simulink model "Timers"  (R2025a)
settings: Solver=FixedStepDiscrete  StartTime=0  StopTime=1  FixedStep=1e-7  RelTol=1e-3
libraries: simulink_extras x216, simulink x13
(part 7 of 7)

== system Timers/Eg: PWM Driver+  Prescalar/Tcon/Subsystem5 ==
  Data : Inport
  Store : Inport  Port=2
  Clock : Inport  Port=3
  Clear : Inport  Port=4
  AND : Logic  IconShape=distinctive  AllPortsSameDT=off  OutDataTypeStr=boolean
  AND1 : Logic  IconShape=distinctive  AllPortsSameDT=off  OutDataTypeStr=boolean
  D Flip-Flop : simulink_extras/Flip Flops/D Flip-Flop
  NOT : Logic  Operator=NOT  IconShape=distinctive  AllPortsSameDT=off  OutDataTypeStr=boolean
  NOT1 : Logic  Operator=NOT  IconShape=distinctive  AllPortsSameDT=off  OutDataTypeStr=boolean
  OR : Logic  Operator=OR  IconShape=distinctive  AllPortsSameDT=off  OutDataTypeStr=boolean
  Q : Outport
  !Q : Outport  Port=2
  wires:
  AND1/1 -> OR/2
  AND/1 -> OR/1
  D Flip-Flop/1 -> Q/1, AND1/2
  NOT/1 -> AND1/1
  Store/1 -> AND/2, NOT/1
  Clock/1 -> D Flip-Flop/2
  Data/1 -> AND/1
  OR/1 -> D Flip-Flop/1
  D Flip-Flop/2 -> !Q/1
  Clear/1 -> NOT1/1
  NOT1/1 -> D Flip-Flop/3

== system Timers/Eg: PWM Driver+  Prescalar/Tcon/Subsystem6 ==
  Data : Inport
  Store : Inport  Port=2
  Clock : Inport  Port=3
  Clear : Inport  Port=4
  AND : Logic  IconShape=distinctive  AllPortsSameDT=off  OutDataTypeStr=boolean
  AND1 : Logic  IconShape=distinctive  AllPortsSameDT=off  OutDataTypeStr=boolean
  D Flip-Flop : simulink_extras/Flip Flops/D Flip-Flop
  NOT : Logic  Operator=NOT  IconShape=distinctive  AllPortsSameDT=off  OutDataTypeStr=boolean
  NOT1 : Logic  Operator=NOT  IconShape=distinctive  AllPortsSameDT=off  OutDataTypeStr=boolean
  OR : Logic  Operator=OR  IconShape=distinctive  AllPortsSameDT=off  OutDataTypeStr=boolean
  Q : Outport
  !Q : Outport  Port=2
  wires:
  AND1/1 -> OR/2
  AND/1 -> OR/1
  D Flip-Flop/1 -> Q/1, AND1/2
  NOT/1 -> AND1/1
  Store/1 -> AND/2, NOT/1
  Clock/1 -> D Flip-Flop/2
  Data/1 -> AND/1
  OR/1 -> D Flip-Flop/1
  D Flip-Flop/2 -> !Q/1
  Clear/1 -> NOT1/1
  NOT1/1 -> D Flip-Flop/3

== system Timers/Eg: PWM Driver+  Prescalar/Tcon/Subsystem7 ==
  Data : Inport
  Store : Inport  Port=2
  Clock : Inport  Port=3
  Clear : Inport  Port=4
  AND : Logic  IconShape=distinctive  AllPortsSameDT=off  OutDataTypeStr=boolean
  AND1 : Logic  IconShape=distinctive  AllPortsSameDT=off  OutDataTypeStr=boolean
  D Flip-Flop : simulink_extras/Flip Flops/D Flip-Flop
  NOT : Logic  Operator=NOT  IconShape=distinctive  AllPortsSameDT=off  OutDataTypeStr=boolean
  NOT1 : Logic  Operator=NOT  IconShape=distinctive  AllPortsSameDT=off  OutDataTypeStr=boolean
  OR : Logic  Operator=OR  IconShape=distinctive  AllPortsSameDT=off  OutDataTypeStr=boolean
  Q : Outport
  !Q : Outport  Port=2
  wires:
  AND1/1 -> OR/2
  AND/1 -> OR/1
  D Flip-Flop/1 -> Q/1, AND1/2
  NOT/1 -> AND1/1
  Store/1 -> AND/2, NOT/1
  Clock/1 -> D Flip-Flop/2
  Data/1 -> AND/1
  OR/1 -> D Flip-Flop/1
  D Flip-Flop/2 -> !Q/1
  Clear/1 -> NOT1/1
  NOT1/1 -> D Flip-Flop/3

== system Timers/Eg: PWM Driver+  Prescalar/Tcon/Subsystem8 ==
  Data : Inport
  Store : Inport  Port=2
  Clock : Inport  Port=3
  Clear : Inport  Port=4
  AND : Logic  IconShape=distinctive  AllPortsSameDT=off  OutDataTypeStr=boolean
  AND1 : Logic  IconShape=distinctive  AllPortsSameDT=off  OutDataTypeStr=boolean
  D Flip-Flop : simulink_extras/Flip Flops/D Flip-Flop
  NOT : Logic  Operator=NOT  IconShape=distinctive  AllPortsSameDT=off  OutDataTypeStr=boolean
  NOT1 : Logic  Operator=NOT  IconShape=distinctive  AllPortsSameDT=off  OutDataTypeStr=boolean
  OR : Logic  Operator=OR  IconShape=distinctive  AllPortsSameDT=off  OutDataTypeStr=boolean
  Q : Outport
  !Q : Outport  Port=2
  wires:
  AND1/1 -> OR/2
  AND/1 -> OR/1
  D Flip-Flop/1 -> Q/1, AND1/2
  NOT/1 -> AND1/1
  Store/1 -> AND/2, NOT/1
  Clock/1 -> D Flip-Flop/2
  Data/1 -> AND/1
  OR/1 -> D Flip-Flop/1
  D Flip-Flop/2 -> !Q/1
  Clear/1 -> NOT1/1
  NOT1/1 -> D Flip-Flop/3

== system Timers/Eg: Prescaler/Counter/Half Adder ==
  A : Inport
  "B " : Inport  Port=2
  AND : Logic  IconShape=distinctive  AllPortsSameDT=off  OutDataTypeStr=boolean
  XOR : Logic  Operator=XOR  IconShape=distinctive  AllPortsSameDT=off  OutDataTypeStr=boolean
  Sum : Outport
  Carry : Outport  Port=2
  wires:
  A/1 -> AND/1, XOR/1
  "B "/1 -> XOR/2, AND/2
  XOR/1 -> Sum/1
  AND/1 -> Carry/1

== system Timers/Eg: Prescaler/Counter/Half Adder1 ==
  A : Inport
  "B " : Inport  Port=2
  AND : Logic  IconShape=distinctive  AllPortsSameDT=off  OutDataTypeStr=boolean
  XOR : Logic  Operator=XOR  IconShape=distinctive  AllPortsSameDT=off  OutDataTypeStr=boolean
  Sum : Outport
  Carry : Outport  Port=2
  wires:
  A/1 -> AND/1, XOR/1
  "B "/1 -> XOR/2, AND/2
  XOR/1 -> Sum/1
  AND/1 -> Carry/1

== system Timers/Eg: Prescaler/Counter/Half Adder2 ==
  A : Inport
  "B " : Inport  Port=2
  AND : Logic  IconShape=distinctive  AllPortsSameDT=off  OutDataTypeStr=boolean
  XOR : Logic  Operator=XOR  IconShape=distinctive  AllPortsSameDT=off  OutDataTypeStr=boolean
  Sum : Outport
  Carry : Outport  Port=2
  wires:
  A/1 -> AND/1, XOR/1
  "B "/1 -> XOR/2, AND/2
  XOR/1 -> Sum/1
  AND/1 -> Carry/1

== system Timers/Eg: Prescaler/Counter/Half Adder3 ==
  A : Inport
  "B " : Inport  Port=2
  AND : Logic  IconShape=distinctive  AllPortsSameDT=off  OutDataTypeStr=boolean
  XOR : Logic  Operator=XOR  IconShape=distinctive  AllPortsSameDT=off  OutDataTypeStr=boolean
  Sum : Outport
  Carry : Outport  Port=2
  wires:
  A/1 -> AND/1, XOR/1
  "B "/1 -> XOR/2, AND/2
  XOR/1 -> Sum/1
  AND/1 -> Carry/1

== system Timers/Eg: Prescaler/Counter/Half Adder4 ==
  A : Inport
  "B " : Inport  Port=2
  AND : Logic  IconShape=distinctive  AllPortsSameDT=off  OutDataTypeStr=boolean
  XOR : Logic  Operator=XOR  IconShape=distinctive  AllPortsSameDT=off  OutDataTypeStr=boolean
  Sum : Outport
  Carry : Outport  Port=2
  wires:
  A/1 -> AND/1, XOR/1
  "B "/1 -> XOR/2, AND/2
  XOR/1 -> Sum/1
  AND/1 -> Carry/1

== system Timers/Eg: Prescaler/Counter/Half Adder5 ==
  A : Inport
  "B " : Inport  Port=2
  AND : Logic  IconShape=distinctive  AllPortsSameDT=off  OutDataTypeStr=boolean
  XOR : Logic  Operator=XOR  IconShape=distinctive  AllPortsSameDT=off  OutDataTypeStr=boolean
  Sum : Outport
  Carry : Outport  Port=2
  wires:
  A/1 -> AND/1, XOR/1
  "B "/1 -> XOR/2, AND/2
  XOR/1 -> Sum/1
  AND/1 -> Carry/1

== system Timers/Eg: Prescaler/Counter/Half Adder6 ==
  A : Inport
  "B " : Inport  Port=2
  XOR : Logic  Operator=XOR  IconShape=distinctive  AllPortsSameDT=off  OutDataTypeStr=boolean
  Sum : Outport
  wires:
  A/1 -> XOR/1
  "B "/1 -> XOR/2
  XOR/1 -> Sum/1

== system Timers/Eg: Prescaler/Counter/Half Adder7 ==
  A : Inport
  "B " : Inport  Port=2
  AND : Logic  IconShape=distinctive  AllPortsSameDT=off  OutDataTypeStr=boolean
  XOR : Logic  Operator=XOR  IconShape=distinctive  AllPortsSameDT=off  OutDataTypeStr=boolean
  Sum : Outport
  Carry : Outport  Port=2
  wires:
  A/1 -> AND/1, XOR/1
  "B "/1 -> XOR/2, AND/2
  XOR/1 -> Sum/1
  AND/1 -> Carry/1

== system Timers/Eg: Prescaler/Counter1/Half Adder ==
  A : Inport
  "B " : Inport  Port=2
  AND : Logic  IconShape=distinctive  AllPortsSameDT=off  OutDataTypeStr=boolean
  XOR : Logic  Operator=XOR  IconShape=distinctive  AllPortsSameDT=off  OutDataTypeStr=boolean
  Sum : Outport
  Carry : Outport  Port=2
  wires:
  A/1 -> AND/1, XOR/1
  "B "/1 -> XOR/2, AND/2
  XOR/1 -> Sum/1
  AND/1 -> Carry/1

== system Timers/Eg: Prescaler/Counter1/Half Adder1 ==
  A : Inport
  "B " : Inport  Port=2
  AND : Logic  IconShape=distinctive  AllPortsSameDT=off  OutDataTypeStr=boolean
  XOR : Logic  Operator=XOR  IconShape=distinctive  AllPortsSameDT=off  OutDataTypeStr=boolean
  Sum : Outport
  Carry : Outport  Port=2
  wires:
  A/1 -> AND/1, XOR/1
  "B "/1 -> XOR/2, AND/2
  XOR/1 -> Sum/1
  AND/1 -> Carry/1

== system Timers/Eg: Prescaler/Counter1/Half Adder2 ==
  A : Inport
  "B " : Inport  Port=2
  AND : Logic  IconShape=distinctive  AllPortsSameDT=off  OutDataTypeStr=boolean
  XOR : Logic  Operator=XOR  IconShape=distinctive  AllPortsSameDT=off  OutDataTypeStr=boolean
  Sum : Outport
  Carry : Outport  Port=2
  wires:
  A/1 -> AND/1, XOR/1
  "B "/1 -> XOR/2, AND/2
  XOR/1 -> Sum/1
  AND/1 -> Carry/1

== system Timers/Eg: Prescaler/Counter1/Half Adder3 ==
  A : Inport
  "B " : Inport  Port=2
  AND : Logic  IconShape=distinctive  AllPortsSameDT=off  OutDataTypeStr=boolean
  XOR : Logic  Operator=XOR  IconShape=distinctive  AllPortsSameDT=off  OutDataTypeStr=boolean
  Sum : Outport
  Carry : Outport  Port=2
  wires:
  A/1 -> AND/1, XOR/1
  "B "/1 -> XOR/2, AND/2
  XOR/1 -> Sum/1
  AND/1 -> Carry/1

== system Timers/Eg: Prescaler/Counter1/Half Adder4 ==
  A : Inport
  "B " : Inport  Port=2
  AND : Logic  IconShape=distinctive  AllPortsSameDT=off  OutDataTypeStr=boolean
  XOR : Logic  Operator=XOR  IconShape=distinctive  AllPortsSameDT=off  OutDataTypeStr=boolean
  Sum : Outport
  Carry : Outport  Port=2
  wires:
  A/1 -> AND/1, XOR/1
  "B "/1 -> XOR/2, AND/2
  XOR/1 -> Sum/1
  AND/1 -> Carry/1

== system Timers/Eg: Prescaler/Counter1/Half Adder5 ==
  A : Inport
  "B " : Inport  Port=2
  AND : Logic  IconShape=distinctive  AllPortsSameDT=off  OutDataTypeStr=boolean
  XOR : Logic  Operator=XOR  IconShape=distinctive  AllPortsSameDT=off  OutDataTypeStr=boolean
  Sum : Outport
  Carry : Outport  Port=2
  wires:
  A/1 -> AND/1, XOR/1
  "B "/1 -> XOR/2, AND/2
  XOR/1 -> Sum/1
  AND/1 -> Carry/1

== system Timers/Eg: Prescaler/Counter1/Half Adder6 ==
  A : Inport
  "B " : Inport  Port=2
  XOR : Logic  Operator=XOR  IconShape=distinctive  AllPortsSameDT=off  OutDataTypeStr=boolean
  Sum : Outport
  wires:
  A/1 -> XOR/1
  "B "/1 -> XOR/2
  XOR/1 -> Sum/1

== system Timers/Eg: Prescaler/Counter1/Half Adder7 ==
  A : Inport
  "B " : Inport  Port=2
  AND : Logic  IconShape=distinctive  AllPortsSameDT=off  OutDataTypeStr=boolean
  XOR : Logic  Operator=XOR  IconShape=distinctive  AllPortsSameDT=off  OutDataTypeStr=boolean
  Sum : Outport
  Carry : Outport  Port=2
  wires:
  A/1 -> AND/1, XOR/1
  "B "/1 -> XOR/2, AND/2
  XOR/1 -> Sum/1
  AND/1 -> Carry/1

== system Timers/Eg: Prescaler/TPS/Subsystem1 ==
  Data : Inport
  Store : Inport  Port=2
  Clock : Inport  Port=3
  Clear : Inport  Port=4
  AND : Logic  IconShape=distinctive  AllPortsSameDT=off  OutDataTypeStr=boolean
  AND1 : Logic  IconShape=distinctive  AllPortsSameDT=off  OutDataTypeStr=boolean
  D Flip-Flop : simulink_extras/Flip Flops/D Flip-Flop
  NOT : Logic  Operator=NOT  IconShape=distinctive  AllPortsSameDT=off  OutDataTypeStr=boolean
  NOT1 : Logic  Operator=NOT  IconShape=distinctive  AllPortsSameDT=off  OutDataTypeStr=boolean
  OR : Logic  Operator=OR  IconShape=distinctive  AllPortsSameDT=off  OutDataTypeStr=boolean
  Q : Outport
  !Q : Outport  Port=2
  wires:
  AND1/1 -> OR/2
  AND/1 -> OR/1
  D Flip-Flop/1 -> Q/1, AND1/2
  NOT/1 -> AND1/1
  Store/1 -> AND/2, NOT/1
  Clock/1 -> D Flip-Flop/2
  Data/1 -> AND/1
  OR/1 -> D Flip-Flop/1
  D Flip-Flop/2 -> !Q/1
  Clear/1 -> NOT1/1
  NOT1/1 -> D Flip-Flop/3

== system Timers/Eg: Prescaler/TPS/Subsystem2 ==
  Data : Inport
  Store : Inport  Port=2
  Clock : Inport  Port=3
  Clear : Inport  Port=4
  AND : Logic  IconShape=distinctive  AllPortsSameDT=off  OutDataTypeStr=boolean
  AND1 : Logic  IconShape=distinctive  AllPortsSameDT=off  OutDataTypeStr=boolean
  D Flip-Flop : simulink_extras/Flip Flops/D Flip-Flop
  NOT : Logic  Operator=NOT  IconShape=distinctive  AllPortsSameDT=off  OutDataTypeStr=boolean
  NOT1 : Logic  Operator=NOT  IconShape=distinctive  AllPortsSameDT=off  OutDataTypeStr=boolean
  OR : Logic  Operator=OR  IconShape=distinctive  AllPortsSameDT=off  OutDataTypeStr=boolean
  Q : Outport
  !Q : Outport  Port=2
  wires:
  AND1/1 -> OR/2
  AND/1 -> OR/1
  D Flip-Flop/1 -> Q/1, AND1/2
  NOT/1 -> AND1/1
  Store/1 -> AND/2, NOT/1
  Clock/1 -> D Flip-Flop/2
  Data/1 -> AND/1
  OR/1 -> D Flip-Flop/1
  D Flip-Flop/2 -> !Q/1
  Clear/1 -> NOT1/1
  NOT1/1 -> D Flip-Flop/3

== system Timers/Eg: Prescaler/TPS/Subsystem3 ==
  Data : Inport
  Store : Inport  Port=2
  Clock : Inport  Port=3
  Clear : Inport  Port=4
  AND : Logic  IconShape=distinctive  AllPortsSameDT=off  OutDataTypeStr=boolean
  AND1 : Logic  IconShape=distinctive  AllPortsSameDT=off  OutDataTypeStr=boolean
  D Flip-Flop : simulink_extras/Flip Flops/D Flip-Flop
  NOT : Logic  Operator=NOT  IconShape=distinctive  AllPortsSameDT=off  OutDataTypeStr=boolean
  NOT1 : Logic  Operator=NOT  IconShape=distinctive  AllPortsSameDT=off  OutDataTypeStr=boolean
  OR : Logic  Operator=OR  IconShape=distinctive  AllPortsSameDT=off  OutDataTypeStr=boolean
  Q : Outport
  !Q : Outport  Port=2
  wires:
  AND1/1 -> OR/2
  AND/1 -> OR/1
  D Flip-Flop/1 -> Q/1, AND1/2
  NOT/1 -> AND1/1
  Store/1 -> AND/2, NOT/1
  Clock/1 -> D Flip-Flop/2
  Data/1 -> AND/1
  OR/1 -> D Flip-Flop/1
  D Flip-Flop/2 -> !Q/1
  Clear/1 -> NOT1/1
  NOT1/1 -> D Flip-Flop/3

== system Timers/Eg: Prescaler/TPS/Subsystem4 ==
  Data : Inport
  Store : Inport  Port=2
  Clock : Inport  Port=3
  Clear : Inport  Port=4
  AND : Logic  IconShape=distinctive  AllPortsSameDT=off  OutDataTypeStr=boolean
  AND1 : Logic  IconShape=distinctive  AllPortsSameDT=off  OutDataTypeStr=boolean
  D Flip-Flop : simulink_extras/Flip Flops/D Flip-Flop
  NOT : Logic  Operator=NOT  IconShape=distinctive  AllPortsSameDT=off  OutDataTypeStr=boolean
  NOT1 : Logic  Operator=NOT  IconShape=distinctive  AllPortsSameDT=off  OutDataTypeStr=boolean
  OR : Logic  Operator=OR  IconShape=distinctive  AllPortsSameDT=off  OutDataTypeStr=boolean
  Q : Outport
  !Q : Outport  Port=2
  wires:
  AND1/1 -> OR/2
  AND/1 -> OR/1
  D Flip-Flop/1 -> Q/1, AND1/2
  NOT/1 -> AND1/1
  Store/1 -> AND/2, NOT/1
  Clock/1 -> D Flip-Flop/2
  Data/1 -> AND/1
  OR/1 -> D Flip-Flop/1
  D Flip-Flop/2 -> !Q/1
  Clear/1 -> NOT1/1
  NOT1/1 -> D Flip-Flop/3

== system Timers/Eg: Prescaler/TPS/Subsystem5 ==
  Data : Inport
  Store : Inport  Port=2
  Clock : Inport  Port=3
  Clear : Inport  Port=4
  AND : Logic  IconShape=distinctive  AllPortsSameDT=off  OutDataTypeStr=boolean
  AND1 : Logic  IconShape=distinctive  AllPortsSameDT=off  OutDataTypeStr=boolean
  D Flip-Flop : simulink_extras/Flip Flops/D Flip-Flop
  NOT : Logic  Operator=NOT  IconShape=distinctive  AllPortsSameDT=off  OutDataTypeStr=boolean
  NOT1 : Logic  Operator=NOT  IconShape=distinctive  AllPortsSameDT=off  OutDataTypeStr=boolean
  OR : Logic  Operator=OR  IconShape=distinctive  AllPortsSameDT=off  OutDataTypeStr=boolean
  Q : Outport
  !Q : Outport  Port=2
  wires:
  AND1/1 -> OR/2
  AND/1 -> OR/1
  D Flip-Flop/1 -> Q/1, AND1/2
  NOT/1 -> AND1/1
  Store/1 -> AND/2, NOT/1
  Clock/1 -> D Flip-Flop/2
  Data/1 -> AND/1
  OR/1 -> D Flip-Flop/1
  D Flip-Flop/2 -> !Q/1
  Clear/1 -> NOT1/1
  NOT1/1 -> D Flip-Flop/3

== system Timers/Eg: Prescaler/TPS/Subsystem6 ==
  Data : Inport
  Store : Inport  Port=2
  Clock : Inport  Port=3
  Clear : Inport  Port=4
  AND : Logic  IconShape=distinctive  AllPortsSameDT=off  OutDataTypeStr=boolean
  AND1 : Logic  IconShape=distinctive  AllPortsSameDT=off  OutDataTypeStr=boolean
  D Flip-Flop : simulink_extras/Flip Flops/D Flip-Flop
  NOT : Logic  Operator=NOT  IconShape=distinctive  AllPortsSameDT=off  OutDataTypeStr=boolean
  NOT1 : Logic  Operator=NOT  IconShape=distinctive  AllPortsSameDT=off  OutDataTypeStr=boolean
  OR : Logic  Operator=OR  IconShape=distinctive  AllPortsSameDT=off  OutDataTypeStr=boolean
  Q : Outport
  !Q : Outport  Port=2
  wires:
  AND1/1 -> OR/2
  AND/1 -> OR/1
  D Flip-Flop/1 -> Q/1, AND1/2
  NOT/1 -> AND1/1
  Store/1 -> AND/2, NOT/1
  Clock/1 -> D Flip-Flop/2
  Data/1 -> AND/1
  OR/1 -> D Flip-Flop/1
  D Flip-Flop/2 -> !Q/1
  Clear/1 -> NOT1/1
  NOT1/1 -> D Flip-Flop/3

== system Timers/Eg: Prescaler/TPS/Subsystem7 ==
  Data : Inport
  Store : Inport  Port=2
  Clock : Inport  Port=3
  Clear : Inport  Port=4
  AND : Logic  IconShape=distinctive  AllPortsSameDT=off  OutDataTypeStr=boolean
  AND1 : Logic  IconShape=distinctive  AllPortsSameDT=off  OutDataTypeStr=boolean
  D Flip-Flop : simulink_extras/Flip Flops/D Flip-Flop
  NOT : Logic  Operator=NOT  IconShape=distinctive  AllPortsSameDT=off  OutDataTypeStr=boolean
  NOT1 : Logic  Operator=NOT  IconShape=distinctive  AllPortsSameDT=off  OutDataTypeStr=boolean
  OR : Logic  Operator=OR  IconShape=distinctive  AllPortsSameDT=off  OutDataTypeStr=boolean
  Q : Outport
  !Q : Outport  Port=2
  wires:
  AND1/1 -> OR/2
  AND/1 -> OR/1
  D Flip-Flop/1 -> Q/1, AND1/2
  NOT/1 -> AND1/1
  Store/1 -> AND/2, NOT/1
  Clock/1 -> D Flip-Flop/2
  Data/1 -> AND/1
  OR/1 -> D Flip-Flop/1
  D Flip-Flop/2 -> !Q/1
  Clear/1 -> NOT1/1
  NOT1/1 -> D Flip-Flop/3

== system Timers/Eg: Prescaler/TPS/Subsystem8 ==
  Data : Inport
  Store : Inport  Port=2
  Clock : Inport  Port=3
  Clear : Inport  Port=4
  AND : Logic  IconShape=distinctive  AllPortsSameDT=off  OutDataTypeStr=boolean
  AND1 : Logic  IconShape=distinctive  AllPortsSameDT=off  OutDataTypeStr=boolean
  D Flip-Flop : simulink_extras/Flip Flops/D Flip-Flop
  NOT : Logic  Operator=NOT  IconShape=distinctive  AllPortsSameDT=off  OutDataTypeStr=boolean
  NOT1 : Logic  Operator=NOT  IconShape=distinctive  AllPortsSameDT=off  OutDataTypeStr=boolean
  OR : Logic  Operator=OR  IconShape=distinctive  AllPortsSameDT=off  OutDataTypeStr=boolean
  Q : Outport
  !Q : Outport  Port=2
  wires:
  AND1/1 -> OR/2
  AND/1 -> OR/1
  D Flip-Flop/1 -> Q/1, AND1/2
  NOT/1 -> AND1/1
  Store/1 -> AND/2, NOT/1
  Clock/1 -> D Flip-Flop/2
  Data/1 -> AND/1
  OR/1 -> D Flip-Flop/1
  D Flip-Flop/2 -> !Q/1
  Clear/1 -> NOT1/1
  NOT1/1 -> D Flip-Flop/3

== system Timers/Eg: Prescaler/TReg/Subsystem1 ==
  Data : Inport
  Store : Inport  Port=2
  Clock : Inport  Port=3
  Clear : Inport  Port=4
  AND : Logic  IconShape=distinctive  AllPortsSameDT=off  OutDataTypeStr=boolean
  AND1 : Logic  IconShape=distinctive  AllPortsSameDT=off  OutDataTypeStr=boolean
  D Flip-Flop : simulink_extras/Flip Flops/D Flip-Flop
  NOT : Logic  Operator=NOT  IconShape=distinctive  AllPortsSameDT=off  OutDataTypeStr=boolean
  NOT1 : Logic  Operator=NOT  IconShape=distinctive  AllPortsSameDT=off  OutDataTypeStr=boolean
  OR : Logic  Operator=OR  IconShape=distinctive  AllPortsSameDT=off  OutDataTypeStr=boolean
  Q : Outport
  !Q : Outport  Port=2
  wires:
  AND1/1 -> OR/2
  AND/1 -> OR/1
  D Flip-Flop/1 -> Q/1, AND1/2
  NOT/1 -> AND1/1
  Store/1 -> AND/2, NOT/1
  Clock/1 -> D Flip-Flop/2
  Data/1 -> AND/1
  OR/1 -> D Flip-Flop/1
  D Flip-Flop/2 -> !Q/1
  Clear/1 -> NOT1/1
  NOT1/1 -> D Flip-Flop/3

== system Timers/Eg: Prescaler/TReg/Subsystem2 ==
  Data : Inport
  Store : Inport  Port=2
  Clock : Inport  Port=3
  Clear : Inport  Port=4
  AND : Logic  IconShape=distinctive  AllPortsSameDT=off  OutDataTypeStr=boolean
  AND1 : Logic  IconShape=distinctive  AllPortsSameDT=off  OutDataTypeStr=boolean
  D Flip-Flop : simulink_extras/Flip Flops/D Flip-Flop
  NOT : Logic  Operator=NOT  IconShape=distinctive  AllPortsSameDT=off  OutDataTypeStr=boolean
  NOT1 : Logic  Operator=NOT  IconShape=distinctive  AllPortsSameDT=off  OutDataTypeStr=boolean
  OR : Logic  Operator=OR  IconShape=distinctive  AllPortsSameDT=off  OutDataTypeStr=boolean
  Q : Outport
  !Q : Outport  Port=2
  wires:
  AND1/1 -> OR/2
  AND/1 -> OR/1
  D Flip-Flop/1 -> Q/1, AND1/2
  NOT/1 -> AND1/1
  Store/1 -> AND/2, NOT/1
  Clock/1 -> D Flip-Flop/2
  Data/1 -> AND/1
  OR/1 -> D Flip-Flop/1
  D Flip-Flop/2 -> !Q/1
  Clear/1 -> NOT1/1
  NOT1/1 -> D Flip-Flop/3

== system Timers/Eg: Prescaler/TReg/Subsystem3 ==
  Data : Inport
  Store : Inport  Port=2
  Clock : Inport  Port=3
  Clear : Inport  Port=4
  AND : Logic  IconShape=distinctive  AllPortsSameDT=off  OutDataTypeStr=boolean
  AND1 : Logic  IconShape=distinctive  AllPortsSameDT=off  OutDataTypeStr=boolean
  D Flip-Flop : simulink_extras/Flip Flops/D Flip-Flop
  NOT : Logic  Operator=NOT  IconShape=distinctive  AllPortsSameDT=off  OutDataTypeStr=boolean
  NOT1 : Logic  Operator=NOT  IconShape=distinctive  AllPortsSameDT=off  OutDataTypeStr=boolean
  OR : Logic  Operator=OR  IconShape=distinctive  AllPortsSameDT=off  OutDataTypeStr=boolean
  Q : Outport
  !Q : Outport  Port=2
  wires:
  AND1/1 -> OR/2
  AND/1 -> OR/1
  D Flip-Flop/1 -> Q/1, AND1/2
  NOT/1 -> AND1/1
  Store/1 -> AND/2, NOT/1
  Clock/1 -> D Flip-Flop/2
  Data/1 -> AND/1
  OR/1 -> D Flip-Flop/1
  D Flip-Flop/2 -> !Q/1
  Clear/1 -> NOT1/1
  NOT1/1 -> D Flip-Flop/3

== system Timers/Eg: Prescaler/TReg/Subsystem4 ==
  Data : Inport
  Store : Inport  Port=2
  Clock : Inport  Port=3
  Clear : Inport  Port=4
  AND : Logic  IconShape=distinctive  AllPortsSameDT=off  OutDataTypeStr=boolean
  AND1 : Logic  IconShape=distinctive  AllPortsSameDT=off  OutDataTypeStr=boolean
  D Flip-Flop : simulink_extras/Flip Flops/D Flip-Flop
  NOT : Logic  Operator=NOT  IconShape=distinctive  AllPortsSameDT=off  OutDataTypeStr=boolean
  NOT1 : Logic  Operator=NOT  IconShape=distinctive  AllPortsSameDT=off  OutDataTypeStr=boolean
  OR : Logic  Operator=OR  IconShape=distinctive  AllPortsSameDT=off  OutDataTypeStr=boolean
  Q : Outport
  !Q : Outport  Port=2
  wires:
  AND1/1 -> OR/2
  AND/1 -> OR/1
  D Flip-Flop/1 -> Q/1, AND1/2
  NOT/1 -> AND1/1
  Store/1 -> AND/2, NOT/1
  Clock/1 -> D Flip-Flop/2
  Data/1 -> AND/1
  OR/1 -> D Flip-Flop/1
  D Flip-Flop/2 -> !Q/1
  Clear/1 -> NOT1/1
  NOT1/1 -> D Flip-Flop/3

== system Timers/Eg: Prescaler/TReg/Subsystem5 ==
  Data : Inport
  Store : Inport  Port=2
  Clock : Inport  Port=3
  Clear : Inport  Port=4
  AND : Logic  IconShape=distinctive  AllPortsSameDT=off  OutDataTypeStr=boolean
  AND1 : Logic  IconShape=distinctive  AllPortsSameDT=off  OutDataTypeStr=boolean
  D Flip-Flop : simulink_extras/Flip Flops/D Flip-Flop
  NOT : Logic  Operator=NOT  IconShape=distinctive  AllPortsSameDT=off  OutDataTypeStr=boolean
  NOT1 : Logic  Operator=NOT  IconShape=distinctive  AllPortsSameDT=off  OutDataTypeStr=boolean
  OR : Logic  Operator=OR  IconShape=distinctive  AllPortsSameDT=off  OutDataTypeStr=boolean
  Q : Outport
  !Q : Outport  Port=2
  wires:
  AND1/1 -> OR/2
  AND/1 -> OR/1
  D Flip-Flop/1 -> Q/1, AND1/2
  NOT/1 -> AND1/1
  Store/1 -> AND/2, NOT/1
  Clock/1 -> D Flip-Flop/2
  Data/1 -> AND/1
  OR/1 -> D Flip-Flop/1
  D Flip-Flop/2 -> !Q/1
  Clear/1 -> NOT1/1
  NOT1/1 -> D Flip-Flop/3

== system Timers/Eg: Prescaler/TReg/Subsystem6 ==
  Data : Inport
  Store : Inport  Port=2
  Clock : Inport  Port=3
  Clear : Inport  Port=4
  AND : Logic  IconShape=distinctive  AllPortsSameDT=off  OutDataTypeStr=boolean
  AND1 : Logic  IconShape=distinctive  AllPortsSameDT=off  OutDataTypeStr=boolean
  D Flip-Flop : simulink_extras/Flip Flops/D Flip-Flop
  NOT : Logic  Operator=NOT  IconShape=distinctive  AllPortsSameDT=off  OutDataTypeStr=boolean
  NOT1 : Logic  Operator=NOT  IconShape=distinctive  AllPortsSameDT=off  OutDataTypeStr=boolean
  OR : Logic  Operator=OR  IconShape=distinctive  AllPortsSameDT=off  OutDataTypeStr=boolean
  Q : Outport
  !Q : Outport  Port=2
  wires:
  AND1/1 -> OR/2
  AND/1 -> OR/1
  D Flip-Flop/1 -> Q/1, AND1/2
  NOT/1 -> AND1/1
  Store/1 -> AND/2, NOT/1
  Clock/1 -> D Flip-Flop/2
  Data/1 -> AND/1
  OR/1 -> D Flip-Flop/1
  D Flip-Flop/2 -> !Q/1
  Clear/1 -> NOT1/1
  NOT1/1 -> D Flip-Flop/3

== system Timers/Eg: Prescaler/TReg/Subsystem7 ==
  Data : Inport
  Store : Inport  Port=2
  Clock : Inport  Port=3
  Clear : Inport  Port=4
  AND : Logic  IconShape=distinctive  AllPortsSameDT=off  OutDataTypeStr=boolean
  AND1 : Logic  IconShape=distinctive  AllPortsSameDT=off  OutDataTypeStr=boolean
  D Flip-Flop : simulink_extras/Flip Flops/D Flip-Flop
  NOT : Logic  Operator=NOT  IconShape=distinctive  AllPortsSameDT=off  OutDataTypeStr=boolean
  NOT1 : Logic  Operator=NOT  IconShape=distinctive  AllPortsSameDT=off  OutDataTypeStr=boolean
  OR : Logic  Operator=OR  IconShape=distinctive  AllPortsSameDT=off  OutDataTypeStr=boolean
  Q : Outport
  !Q : Outport  Port=2
  wires:
  AND1/1 -> OR/2
  AND/1 -> OR/1
  D Flip-Flop/1 -> Q/1, AND1/2
  NOT/1 -> AND1/1
  Store/1 -> AND/2, NOT/1
  Clock/1 -> D Flip-Flop/2
  Data/1 -> AND/1
  OR/1 -> D Flip-Flop/1
  D Flip-Flop/2 -> !Q/1
  Clear/1 -> NOT1/1
  NOT1/1 -> D Flip-Flop/3

== system Timers/Eg: Prescaler/TReg/Subsystem8 ==
  Data : Inport
  Store : Inport  Port=2
  Clock : Inport  Port=3
  Clear : Inport  Port=4
  AND : Logic  IconShape=distinctive  AllPortsSameDT=off  OutDataTypeStr=boolean
  AND1 : Logic  IconShape=distinctive  AllPortsSameDT=off  OutDataTypeStr=boolean
  D Flip-Flop : simulink_extras/Flip Flops/D Flip-Flop
  NOT : Logic  Operator=NOT  IconShape=distinctive  AllPortsSameDT=off  OutDataTypeStr=boolean
  NOT1 : Logic  Operator=NOT  IconShape=distinctive  AllPortsSameDT=off  OutDataTypeStr=boolean
  OR : Logic  Operator=OR  IconShape=distinctive  AllPortsSameDT=off  OutDataTypeStr=boolean
  Q : Outport
  !Q : Outport  Port=2
  wires:
  AND1/1 -> OR/2
  AND/1 -> OR/1
  D Flip-Flop/1 -> Q/1, AND1/2
  NOT/1 -> AND1/1
  Store/1 -> AND/2, NOT/1
  Clock/1 -> D Flip-Flop/2
  Data/1 -> AND/1
  OR/1 -> D Flip-Flop/1
  D Flip-Flop/2 -> !Q/1
  Clear/1 -> NOT1/1
  NOT1/1 -> D Flip-Flop/3

== system Timers/Eg: Prescaler/Tcon/Subsystem1 ==
  Data : Inport
  Store : Inport  Port=2
  Clock : Inport  Port=3
  Clear : Inport  Port=4
  AND : Logic  IconShape=distinctive  AllPortsSameDT=off  OutDataTypeStr=boolean
  AND1 : Logic  IconShape=distinctive  AllPortsSameDT=off  OutDataTypeStr=boolean
  D Flip-Flop : simulink_extras/Flip Flops/D Flip-Flop
  NOT : Logic  Operator=NOT  IconShape=distinctive  AllPortsSameDT=off  OutDataTypeStr=boolean
  NOT1 : Logic  Operator=NOT  IconShape=distinctive  AllPortsSameDT=off  OutDataTypeStr=boolean
  OR : Logic  Operator=OR  IconShape=distinctive  AllPortsSameDT=off  OutDataTypeStr=boolean
  Q : Outport
  !Q : Outport  Port=2
  wires:
  AND1/1 -> OR/2
  AND/1 -> OR/1
  D Flip-Flop/1 -> Q/1, AND1/2
  NOT/1 -> AND1/1
  Store/1 -> AND/2, NOT/1
  Clock/1 -> D Flip-Flop/2
  Data/1 -> AND/1
  OR/1 -> D Flip-Flop/1
  D Flip-Flop/2 -> !Q/1
  Clear/1 -> NOT1/1
  NOT1/1 -> D Flip-Flop/3

== system Timers/Eg: Prescaler/Tcon/Subsystem2 ==
  Data : Inport
  Store : Inport  Port=2
  Clock : Inport  Port=3
  Clear : Inport  Port=4
  AND : Logic  IconShape=distinctive  AllPortsSameDT=off  OutDataTypeStr=boolean
  AND1 : Logic  IconShape=distinctive  AllPortsSameDT=off  OutDataTypeStr=boolean
  D Flip-Flop : simulink_extras/Flip Flops/D Flip-Flop
  NOT : Logic  Operator=NOT  IconShape=distinctive  AllPortsSameDT=off  OutDataTypeStr=boolean
  NOT1 : Logic  Operator=NOT  IconShape=distinctive  AllPortsSameDT=off  OutDataTypeStr=boolean
  OR : Logic  Operator=OR  IconShape=distinctive  AllPortsSameDT=off  OutDataTypeStr=boolean
  Q : Outport
  !Q : Outport  Port=2
  wires:
  AND1/1 -> OR/2
  AND/1 -> OR/1
  D Flip-Flop/1 -> Q/1, AND1/2
  NOT/1 -> AND1/1
  Store/1 -> AND/2, NOT/1
  Clock/1 -> D Flip-Flop/2
  Data/1 -> AND/1
  OR/1 -> D Flip-Flop/1
  D Flip-Flop/2 -> !Q/1
  Clear/1 -> NOT1/1
  NOT1/1 -> D Flip-Flop/3

== system Timers/Eg: Prescaler/Tcon/Subsystem3 ==
  Data : Inport
  Store : Inport  Port=2
  Clock : Inport  Port=3
  Clear : Inport  Port=4
  AND : Logic  IconShape=distinctive  AllPortsSameDT=off  OutDataTypeStr=boolean
  AND1 : Logic  IconShape=distinctive  AllPortsSameDT=off  OutDataTypeStr=boolean
  D Flip-Flop : simulink_extras/Flip Flops/D Flip-Flop
  NOT : Logic  Operator=NOT  IconShape=distinctive  AllPortsSameDT=off  OutDataTypeStr=boolean
  NOT1 : Logic  Operator=NOT  IconShape=distinctive  AllPortsSameDT=off  OutDataTypeStr=boolean
  OR : Logic  Operator=OR  IconShape=distinctive  AllPortsSameDT=off  OutDataTypeStr=boolean
  Q : Outport
  !Q : Outport  Port=2
  wires:
  AND1/1 -> OR/2
  AND/1 -> OR/1
  D Flip-Flop/1 -> Q/1, AND1/2
  NOT/1 -> AND1/1
  Store/1 -> AND/2, NOT/1
  Clock/1 -> D Flip-Flop/2
  Data/1 -> AND/1
  OR/1 -> D Flip-Flop/1
  D Flip-Flop/2 -> !Q/1
  Clear/1 -> NOT1/1
  NOT1/1 -> D Flip-Flop/3

== system Timers/Eg: Prescaler/Tcon/Subsystem4 ==
  Data : Inport
  Store : Inport  Port=2
  Clock : Inport  Port=3
  Clear : Inport  Port=4
  AND : Logic  IconShape=distinctive  AllPortsSameDT=off  OutDataTypeStr=boolean
  AND1 : Logic  IconShape=distinctive  AllPortsSameDT=off  OutDataTypeStr=boolean
  D Flip-Flop : simulink_extras/Flip Flops/D Flip-Flop
  NOT : Logic  Operator=NOT  IconShape=distinctive  AllPortsSameDT=off  OutDataTypeStr=boolean
  NOT1 : Logic  Operator=NOT  IconShape=distinctive  AllPortsSameDT=off  OutDataTypeStr=boolean
  OR : Logic  Operator=OR  IconShape=distinctive  AllPortsSameDT=off  OutDataTypeStr=boolean
  Q : Outport
  !Q : Outport  Port=2
  wires:
  AND1/1 -> OR/2
  AND/1 -> OR/1
  D Flip-Flop/1 -> Q/1, AND1/2
  NOT/1 -> AND1/1
  Store/1 -> AND/2, NOT/1
  Clock/1 -> D Flip-Flop/2
  Data/1 -> AND/1
  OR/1 -> D Flip-Flop/1
  D Flip-Flop/2 -> !Q/1
  Clear/1 -> NOT1/1
  NOT1/1 -> D Flip-Flop/3

== system Timers/Eg: Prescaler/Tcon/Subsystem5 ==
  Data : Inport
  Store : Inport  Port=2
  Clock : Inport  Port=3
  Clear : Inport  Port=4
  AND : Logic  IconShape=distinctive  AllPortsSameDT=off  OutDataTypeStr=boolean
  AND1 : Logic  IconShape=distinctive  AllPortsSameDT=off  OutDataTypeStr=boolean
  D Flip-Flop : simulink_extras/Flip Flops/D Flip-Flop
  NOT : Logic  Operator=NOT  IconShape=distinctive  AllPortsSameDT=off  OutDataTypeStr=boolean
  NOT1 : Logic  Operator=NOT  IconShape=distinctive  AllPortsSameDT=off  OutDataTypeStr=boolean
  OR : Logic  Operator=OR  IconShape=distinctive  AllPortsSameDT=off  OutDataTypeStr=boolean
  Q : Outport
  !Q : Outport  Port=2
  wires:
  AND1/1 -> OR/2
  AND/1 -> OR/1
  D Flip-Flop/1 -> Q/1, AND1/2
  NOT/1 -> AND1/1
  Store/1 -> AND/2, NOT/1
  Clock/1 -> D Flip-Flop/2
  Data/1 -> AND/1
  OR/1 -> D Flip-Flop/1
  D Flip-Flop/2 -> !Q/1
  Clear/1 -> NOT1/1
  NOT1/1 -> D Flip-Flop/3

== system Timers/Eg: Prescaler/Tcon/Subsystem6 ==
  Data : Inport
  Store : Inport  Port=2
  Clock : Inport  Port=3
  Clear : Inport  Port=4
  AND : Logic  IconShape=distinctive  AllPortsSameDT=off  OutDataTypeStr=boolean
  AND1 : Logic  IconShape=distinctive  AllPortsSameDT=off  OutDataTypeStr=boolean
  D Flip-Flop : simulink_extras/Flip Flops/D Flip-Flop
  NOT : Logic  Operator=NOT  IconShape=distinctive  AllPortsSameDT=off  OutDataTypeStr=boolean
  NOT1 : Logic  Operator=NOT  IconShape=distinctive  AllPortsSameDT=off  OutDataTypeStr=boolean
  OR : Logic  Operator=OR  IconShape=distinctive  AllPortsSameDT=off  OutDataTypeStr=boolean
  Q : Outport
  !Q : Outport  Port=2
  wires:
  AND1/1 -> OR/2
  AND/1 -> OR/1
  D Flip-Flop/1 -> Q/1, AND1/2
  NOT/1 -> AND1/1
  Store/1 -> AND/2, NOT/1
  Clock/1 -> D Flip-Flop/2
  Data/1 -> AND/1
  OR/1 -> D Flip-Flop/1
  D Flip-Flop/2 -> !Q/1
  Clear/1 -> NOT1/1
  NOT1/1 -> D Flip-Flop/3

== system Timers/Eg: Prescaler/Tcon/Subsystem7 ==
  Data : Inport
  Store : Inport  Port=2
  Clock : Inport  Port=3
  Clear : Inport  Port=4
  AND : Logic  IconShape=distinctive  AllPortsSameDT=off  OutDataTypeStr=boolean
  AND1 : Logic  IconShape=distinctive  AllPortsSameDT=off  OutDataTypeStr=boolean
  D Flip-Flop : simulink_extras/Flip Flops/D Flip-Flop
  NOT : Logic  Operator=NOT  IconShape=distinctive  AllPortsSameDT=off  OutDataTypeStr=boolean
  NOT1 : Logic  Operator=NOT  IconShape=distinctive  AllPortsSameDT=off  OutDataTypeStr=boolean
  OR : Logic  Operator=OR  IconShape=distinctive  AllPortsSameDT=off  OutDataTypeStr=boolean
  Q : Outport
  !Q : Outport  Port=2
  wires:
  AND1/1 -> OR/2
  AND/1 -> OR/1
  D Flip-Flop/1 -> Q/1, AND1/2
  NOT/1 -> AND1/1
  Store/1 -> AND/2, NOT/1
  Clock/1 -> D Flip-Flop/2
  Data/1 -> AND/1
  OR/1 -> D Flip-Flop/1
  D Flip-Flop/2 -> !Q/1
  Clear/1 -> NOT1/1
  NOT1/1 -> D Flip-Flop/3

== system Timers/Eg: Prescaler/Tcon/Subsystem8 ==
  Data : Inport
  Store : Inport  Port=2
  Clock : Inport  Port=3
  Clear : Inport  Port=4
  AND : Logic  IconShape=distinctive  AllPortsSameDT=off  OutDataTypeStr=boolean
  AND1 : Logic  IconShape=distinctive  AllPortsSameDT=off  OutDataTypeStr=boolean
  D Flip-Flop : simulink_extras/Flip Flops/D Flip-Flop
  NOT : Logic  Operator=NOT  IconShape=distinctive  AllPortsSameDT=off  OutDataTypeStr=boolean
  NOT1 : Logic  Operator=NOT  IconShape=distinctive  AllPortsSameDT=off  OutDataTypeStr=boolean
  OR : Logic  Operator=OR  IconShape=distinctive  AllPortsSameDT=off  OutDataTypeStr=boolean
  Q : Outport
  !Q : Outport  Port=2
  wires:
  AND1/1 -> OR/2
  AND/1 -> OR/1
  D Flip-Flop/1 -> Q/1, AND1/2
  NOT/1 -> AND1/1
  Store/1 -> AND/2, NOT/1
  Clock/1 -> D Flip-Flop/2
  Data/1 -> AND/1
  OR/1 -> D Flip-Flop/1
  D Flip-Flop/2 -> !Q/1
  Clear/1 -> NOT1/1
  NOT1/1 -> D Flip-Flop/3

== stateflow chart Timers/Chart2 ==
  state Load_TH
    entry:
    CLR=0;
    Data = TH
    StoreTH=1;
  state Startup
    entry:
    Data= 0;
  state wait
    entry:
    StoreTH=0;
  state Load_TL
    entry:
    CLR=0;
    Data = TL
    StoreTL=1;
  state wait3
    entry:
    StoreTL=0;
  state END
    entry:
    StoreTCON=0;
    Data=0;
  state Load_TCON
    entry:
    Data=TCON;
    StoreTCON=1;
  state wait2
    entry:
    StoreTPS=0;
  state Load_TPS
    entry:
    Data=TPS;
    StoreTPS=1;
  (default) -> Startup
  Startup -> Load_TH : [Start==1&&CLK==0]
  END -> Startup : [Start==0]
  Load_TH -> wait : [CLK==1]
  wait -> Load_TL : [CLK==0]
  Load_TL -> wait3 : [CLK==1]
  wait3 -> Load_TPS : [CLK==0]
  Load_TCON -> END : [CLK==1]
  wait2 -> Load_TCON : [CLK==0]
  Load_TPS -> wait2 : [CLK==1]
  data: TCON input; Start input; CLR output; Data output; StoreTPS output; CLK input; TH input; StoreTCON output; TPS input; StoreTH output; StoreTL output; TL input

== matlab function Timers/Subsystem/MATLAB Function ==
  data: number input; a output; b output; c output; d output; e output; f output; g output; h output
function [a, b, c, d, e, f, g, h] = numToBinary8BitOutputs(number)
    % Initialise the Signed output

    % Ensure the input is within the valid range for unsigned numbers (0 to 255)
    if number < 0
        % For signed mode, enable Signed flag and check if the number is >= -128
        if number < -128
            % If below -128, set all outputs to 0
            [a, b, c, d, e, f, g, h] = deal(false, false, false, false, false, false, false, false);
            return;
        else
            % Convert the number to 2's complement representation
            number = 256 + number; % Adjust to positive equivalent for 2's complement
        end
    elseif number > 255
        % If outside the unsigned range, set all outputs to 0
        [a, b, c, d, e, f, g, h] = deal(false, false, false, false, false, false, false, false);
        return;
    end

    % Convert the number to an 8-bit binary using manual calculation
    a = logical(mod(floor(number / 128), 2));
    b = logical(mod(floor(number / 64), 2));
    c = logical(mod(floor(number / 32), 2));
    d = logical(mod(floor(number / 16), 2));
    e = logical(mod(floor(number / 8), 2));
    f = logical(mod(floor(number / 4), 2));
    g = logical(mod(floor(number / 2), 2));
    h = logical(mod(number, 2));
end

== matlab function Timers/MATLAB Function2 ==
  data: Binary input; Decimal output
function Decimal = fcn(Binary)
    % Ensure the input is an 8-bit signal
    assert(length(Binary) == 8, 'Input must be an 8-bit binary signal');
    % Convert the logical array (true/false) to a double array (1/0)
    Binary = double(Binary);
    % Calculate the decimal value
    Decimal = 0;
    for i = 1:8
        Decimal = Decimal + Binary(i) * 2^(8 - i);
    end
end

== matlab function Timers/MATLAB Function1 ==
  data: Binary input; Decimal output
function Decimal = fcn(Binary)
    % Ensure the input is an 8-bit signal
    assert(length(Binary) == 8, 'Input must be an 8-bit binary signal');
    % Convert the logical array (true/false) to a double array (1/0)
    Binary = double(Binary);
    % Calculate the decimal value
    Decimal = 0;
    for i = 1:8
        Decimal = Decimal + Binary(i) * 2^(8 - i);
    end
end

== matlab function Timers/MATLAB Function3 ==
  data: Binary input; Decimal output
function Decimal = fcn(Binary)
    % Ensure the input is an 8-bit signal
    assert(length(Binary) == 8, 'Input must be an 8-bit binary signal');
    % Convert the logical array (true/false) to a double array (1/0)
    Binary = double(Binary);
    % Calculate the decimal value
    Decimal = 0;
    for i = 1:8
        Decimal = Decimal + Binary(i) * 2^(8 - i);
    end
end

== stateflow chart Timers/Chart ==
  state Startup
    entry:
    Data= 0;
  state Load_TReg
    entry:
    CLR=0;
    Data = TReg
    StoreTreg=1;
  state Wait1
  state wait
    entry:
    StoreTreg=0;
  state Wait2
  state END
    StoreTCON=0;
  state Load_TCON
    entry:
    Data=TCON;
    StoreTCON=1;
  state Wait3
  (default) -> Startup
  Startup -> Load_TReg : [Start==1&&CLK==0]
  Load_TReg -> Wait1 : [CLK==1]
  END -> Startup : [Start == 0]
  Wait1 -> wait : [CLK==0]
  wait -> Wait2 : [CLK==1]
  Wait2 -> Load_TCON : [CLK==0]
  Wait3 -> END : [CLK==1]
  Load_TCON -> Wait3 : [CLK==0]
  data: TCON input; Start input; CLR output; Data output; CLK input; StoreTreg output; TReg input; StoreTCON output

== stateflow chart Timers/Chart1 ==
  state Load_TReg
    entry:
    CLR=0;
    Data = TReg
    StoreTreg=1;
  state Startup
    entry:
    Data= 0;
  state wait
    entry:
    StoreTreg=0;
  state END
    entry:
    StoreTCON=0;
    Data=0;
  state Load_TCON
    entry:
    Data=TCON;
    StoreTCON=1;
  state wait2
    entry:
    StoreTPS=0;
  state Load_TPS
    entry:
    Data=TPS;
    StoreTPS=1;
  (default) -> Startup
  Startup -> Load_TReg : [Start==1&&CLK==0]
  END -> Startup : [Start==0]
  Load_TReg -> wait : [CLK==1]
  wait -> Load_TPS : [CLK==0]
  Load_TCON -> END : [CLK==1]
  wait2 -> Load_TCON : [CLK==0]
  Load_TPS -> wait2 : [CLK==1]
  data: TCON input; Start input; CLR output; Data output; StoreTPS output; CLK input; StoreTreg output; TReg input; StoreTCON output; TPS input
